simulink model "Energy_management_controller"  (R2014a)
settings: Solver=ode45  SolverMode=SingleTasking  StartTime=0.0  StopTime=10.0  RelTol=1e-3
libraries: fuzblock x1
(part 1 of 2)
settings Model: Creator=12730  LastModifiedBy=Administrator
settings OptimizationCC: BlockReduction=off  BooleanDataType=off  SimCompilerOptimization=off
settings DebuggingCC: SaveWithParameterizedLinksMsg=none  UnderspecifiedInitializationDetection=Classic  SignalResolutionControl=TryResolveAllWithWarning  SolverPrmCheckMsg=none  FrameProcessingCompatibilityMsg=error  StrictBusMsg=Warning
settings HardwareCC: TargetUnknown=on
settings RTWCC: RTWCompilerOptimization=off
settings ConfigComp: CovMetricSettings=dw  CovHtmlReporting=on  CovSaveCumulativeToWorkspaceVar=on  CovSaveSingleToWorkspaceVar=on  CovModelRefEnable=Off  CovExternalEMLEnable=off  CovSFcnEnable=off

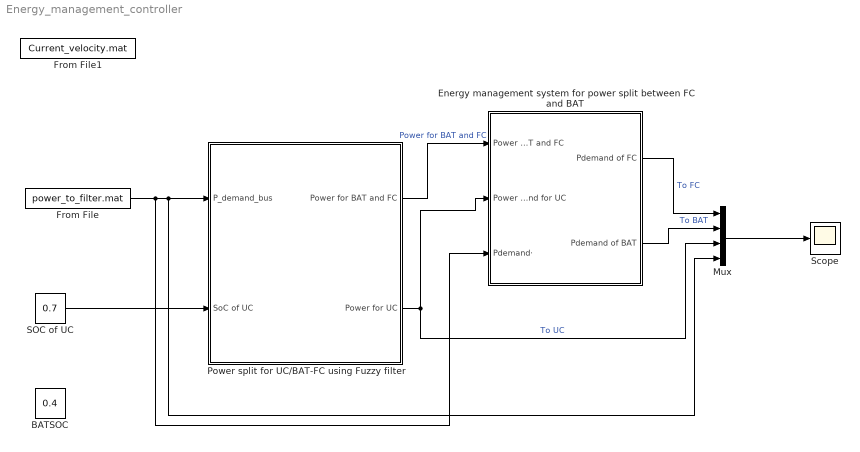
== system Energy_management_controller ==
  "BATSOC " : Constant  Value=0.4
  Energy management system for power split between FC and BAT : Subsystem
  From File : FromFile  FileName=power_to_filter.mat  SampleTime=0
  From File1 : FromFile  FileName=Current_velocity.mat  SampleTime=0
  Mux : Mux
  Power split for UC/BAT-FC using Fuzzy filter : Subsystem
  SOC of UC : Constant  Value=0.7
  Scope : Scope
  wires:
  From File/1 -> Power split for UC/BAT-FC using Fuzzy filter/1(P_demand_bus), Mux/4, Energy management system for power split between FC and BAT/3(Pdemand·)
  Power split for UC/BAT-FC using Fuzzy filter/1(Power for BAT and FC) -> Energy management system for power split between FC and BAT/1(Power demand for BAT and FC)  "Power for BAT and FC"
  Energy management system for power split between FC and BAT/2(Pdemand of BAT) -> Mux/2  "To BAT"
  Power split for UC/BAT-FC using Fuzzy filter/2(Power for UC) -> Energy management system for power split between FC and BAT/2(Power demand for UC), Mux/3  "To UC"
  SOC of UC/1 -> Power split for UC/BAT-FC using Fuzzy filter/2(SoC of UC)
  Mux/1 -> Scope/1
  Energy management system for power split between FC and BAT/1(Pdemand of FC) -> Mux/1  "To FC"

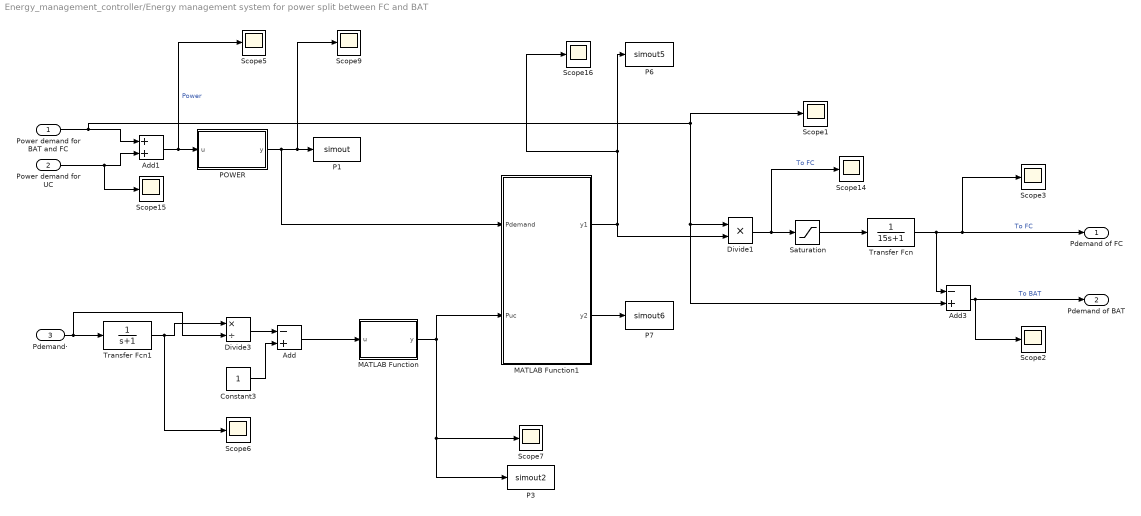
== system Energy_management_controller/Energy management system for power split between FC and BAT ==
  Power demand for BAT and FC : Inport
  Power demand for UC : Inport  Port=2
  Pdemand· : Inport  Port=3
  Add : Sum  Inputs=-+
  Add1 : Sum
  Add3 : Sum  Inputs=-+
  Constant3 : Constant
  Divide1 : Product  Inputs=**
  Divide3 : Product  Inputs=*/
  MATLAB Function : MATLAB Function  TreatAsAtomicUnit=on
  MATLAB Function1 : MATLAB Function  TreatAsAtomicUnit=on
  P1 : ToWorkspace  VariableName=simout  SaveFormat=Timeseries  SampleTime=-1
  P3 : ToWorkspace  VariableName=simout2  SaveFormat=Timeseries  SampleTime=-1
  P6 : ToWorkspace  VariableName=simout5  SaveFormat=Timeseries  SampleTime=-1
  P7 : ToWorkspace  VariableName=simout6  SaveFormat=Timeseries  SampleTime=-1
  POWER : MATLAB Function  TreatAsAtomicUnit=on
  Saturation : Saturate  UpperLimit=10000  LowerLimit=0.5
  Scope{1..3,5..7,9,14..16} (10 alike) : Scope
      Scope7 settings: SaveName=ScopeData3
  Transfer Fcn : TransferFcn  Denominator=[15 1]
  Transfer Fcn1 : TransferFcn  Denominator=[1 1]
  Pdemand of FC : Outport
  Pdemand of BAT : Outport  Port=2
  wires:
  Power demand for UC/1 -> Scope15/1, Add1/2
  Add1/1 -> POWER/1(u), Scope5/1  "Power"
  Add3/1 -> Scope2/1, Pdemand of BAT/1  "To BAT"
  Transfer Fcn/1 -> Add3/1, Pdemand of FC/1, Scope3/1  "To FC"
  Divide1/1 -> Scope14/1, Saturation/1  "To FC"
  Saturation/1 -> Transfer Fcn/1
  Pdemand·/1 -> Transfer Fcn1/1, Divide3/2
  Transfer Fcn1/1 -> Scope6/1, Divide3/1
  Divide3/1 -> Add/1
  Add/1 -> MATLAB Function/1(u)
  Constant3/1 -> Add/2
  MATLAB Function/1(y) -> P3/1, Scope7/1, MATLAB Function1/2(Puc)
  Power demand for BAT and FC/1 -> Add1/1, Add3/2, Divide1/1, Scope1/1
  MATLAB Function1/1(y1) -> Divide1/2, P6/1, Scope16/1
  MATLAB Function1/2(y2) -> P7/1
  POWER/1(y) -> MATLAB Function1/1(Pdemand), P1/1, Scope9/1

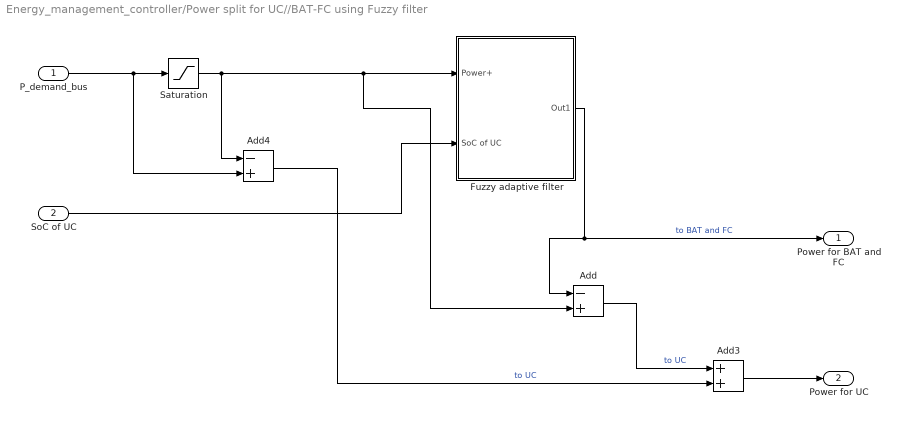
== system Energy_management_controller/Power split for UC//BAT-FC using Fuzzy filter ==
  P_demand_bus : Inport
  SoC of UC : Inport  Port=2
  Add : Sum  Inputs=-+
  Add3 : Sum
  Add4 : Sum  Inputs=-+
  Fuzzy adaptive filter : Subsystem
  Saturation : Saturate  UpperLimit=100000  LowerLimit=0
  Power for BAT and FC : Outport
  Power for UC : Outport  Port=2
  wires:
  SoC of UC/1 -> Fuzzy adaptive filter/2(SoC of UC)
  Fuzzy adaptive filter/1(Out1) -> Power for BAT and FC/1, Add/1  "to BAT and FC"
  P_demand_bus/1 -> Saturation/1, Add4/2
  Add/1 -> Add3/1  "to UC"
  Add4/1 -> Add3/2  "to UC"
  Add3/1 -> Power for UC/1
  Saturation/1 -> Add/2, Fuzzy adaptive filter/1(Power+), Add4/1

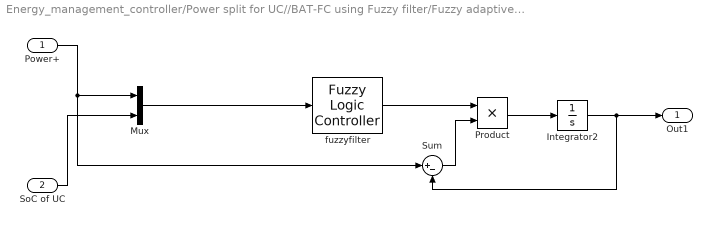
== system Energy_management_controller/Power split for UC//BAT-FC using Fuzzy filter/Fuzzy adaptive filter ==
  Power+ : Inport
  SoC of UC : Inport  Port=2
  Integrator2 : Integrator
  Mux : Mux  Inputs=2
  Product : Product
  Sum : Sum  Inputs=|+-
  fuzzyfilter : fuzblock/Fuzzy Logic  Controller  fis=['fuzzyfilter1']
  Out1 : Outport
  wires:
  Power+/1 -> Sum/1, Mux/1
  fuzzyfilter/1 -> Product/1
  Sum/1 -> Product/2
  Product/1 -> Integrator2/1
  Integrator2/1 -> Out1/1, Sum/2
  SoC of UC/1 -> Mux/2
  Mux/1 -> fuzzyfilter/1

== matlab function Energy_management_controller/Energy management system for power split between FC and BAT/MATLAB Function2 ==
  data: u input; y output
function y = fcn(u)
%#codegen

y = u;

== matlab function Energy_management_controller/Energy management system for power split between FC and BAT/POWER ==
  data: u input; y output
function y = fcn(u)
            n = floor(u);
            m = u - n;
            
     if m >= 0.25 &&m < 0.75
            m = 0.5;
            u = n + m;
        else if m < 0.25&& 0 <= m
            m = 0;
            u = n + m;
            else 
             m = 0;
             u = n + m + 1;
            end
      end
y = u;

== matlab function Energy_management_controller/Energy management system for power split between FC and BAT/MATLAB Function1 ==
  data: y1 output; Pdemand input; Puc input; y2 output
function [y1,y2] = fcn(Pdemand,Puc)

if Puc==0&&Pdemand>=0

    if Pdemand<=2.5
        P_FC = 0.1;
        P_BAT = 0.9;
        else if Pdemand>=3&&Pdemand<=9
            P_FC = 1;
            P_BAT = 0;
            else if Pdemand>=9.5&&Pdemand<=10
                P_FC = 0.95;
                P_BAT = 0.05;
                else if Pdemand>=10.5&&Pdemand<=12
                        P_FC = 0.65;
                        P_BAT = 0.35;
                    else if Pdemand>=12.5&&Pdemand<=14
                          P_FC = 0.6;
                        P_BAT = 0.4;
                        else if Pdemand>=14.5&&Pdemand<=15
                                  P_FC = 0.5;
                                P_BAT = 0.5;
                               else if Pdemand>=15.5&&Pdemand<=18.5
                                         P_FC = 0.4;
                                         P_BAT = 0.6;
%                                     else if Pdemand>=14.5&&Pdemand<=15
%                                           P_FC = 0.5;
%                                         P_BAT = 0.5;
%                                         else if Pdemand>=15&&Pdemand<=22.5
%                                                   P_FC = 0.5;
%                                                 P_BAT = 0.5;
                                            else 
                                                      P_FC = 0.35;
                                                    P_BAT = 0.65;
%                                          end
%                                         end
                                   end
                              end
                          end
                      end
                 end
            end
    end
else if Puc==0.2&&Pdemand>=0  
         
        if Pdemand>=0.5&&Pdemand<=4
                    P_FC = 0.2;
                    P_BAT = 0.8;
                else if Pdemand>=4.5&&Pdemand<=8.5
                            P_FC = 0.8;
                            P_BAT = 0.2;
                    else if Pdemand>=9&&Pdemand<=10
                                P_FC = 0.75;
                                P_BAT = 0.25;
                        else if Pdemand>=10.5&&Pdemand<=12
                                    P_FC = 0.5;
                                    P_BAT = 0.5;
                            else if Pdemand>=12.5&&Pdemand<=14
                                          P_FC = 0.55;
                                          P_BAT = 0.55;
                                else if Pdemand>=14.5&&Pdemand<=15
                                              P_FC = 0.45;
                                              P_BAT = 0.55;
                                       else if Pdemand>=15.5&&Pdemand<=18.5
                                                P_FC = 0.4;
                                                P_BAT = 0.6;
%                                             else if Pdemand>=12&&Pdemand<=14.5
%                                                       P_FC = 0.7;
%                                                       P_BAT = 0.3;
%                                                 else if Pdemand>=15&&Pdemand<=22.5
%                                                           P_FC = 0.5;
%                                                           P_BAT = 0.5;
                                                      else 
                                                              P_FC = 0.4;
                                                              P_BAT = 0.6;
%                                                     end
%                                                 end
                                           end
                                      end
                                  end
                              end
                         end
                    end
        end  
 else if Puc==0.4&&Pdemand>=0  
         
        if Pdemand>=0.5&&Pdemand<=5.5
                    P_FC = 0.1;
                    P_BAT = 0.9;
                else if Pdemand>=6&&Pdemand<=9
                            P_FC = 0.25;
                            P_BAT = 0.75;
                    else if Pdemand>=9.5&&Pdemand<=10.5
                                P_FC = 0.5;
                                P_BAT = 0.5;
                        else if Pdemand>=11&&Pdemand<=12
                                    P_FC = 0.3;
                                    P_BAT = 0.7;
                            else if Pdemand>=12.5&&Pdemand<=15
                                          P_FC = 0.45;
                                          P_BAT = 0.55;
                                else if Pdemand>=15.5&&Pdemand<=18.5
                                              P_FC = 0.4;
                                              P_BAT = 0.6;
%                                        else if Pdemand>=11&&Pdemand<=11.5
%                                                 P_FC = 0.8;
%                                                 P_BAT = 0.2;
%                                             else if Pdemand>=12&&Pdemand<=14.5
%                                                       P_FC = 0.7;
%                                                       P_BAT = 0.3;
%                                                 else if Pdemand>=15&&Pdemand<=22.5
%                                                           P_FC = 0.5;
%                                                           P_BAT = 0.5;
                                                      else 
                                                              P_FC = 0.35;
                                                              P_BAT = 0.65;
%                                                     end
%                                                 end
%                                            end
                                      end
                                  end
                              end
                         end
                    end
       end  
else if Puc==0.6&&Pdemand>=0  
         
        if Pdemand>=0.5&&Pdemand<=5.5
                    P_FC = 0.1;
                    P_BAT = 0.9;
                else if Pdemand>=6&&Pdemand<=9
                            P_FC = 0.25;
                            P_BAT = 0.75;
                    else if Pdemand>=9.5&&Pdemand<=10.5
                                P_FC = 0.35;
                                P_BAT = 0.65;
                        else if Pdemand>=11&&Pdemand<=12
                                    P_FC = 0.25;
                                    P_BAT = 0.75;
                            else if Pdemand>=12.5&&Pdemand<=18.5
                                          P_FC = 0.4;
                                          P_BAT = 0.6;
%                                 else if Pdemand>=15&&Pdemand<=22.5
%                                               P_FC = 0.5;
%                                               P_BAT = 0.5;
%                                        else if Pdemand>=11&&Pdemand<=11.5
%                                                 P_FC = 0.8;
%                                                 P_BAT = 0.2;
%                                             else if Pdemand>=12&&Pdemand<=14.5
%                                                       P_FC = 0.7;
%                                                       P_BAT = 0.3;
%                                                 else if Pdemand>=15&&Pdemand<=22.5
%                                                           P_FC = 0.5;
%                                                           P_BAT = 0.5;
                                                      else 
                                                              P_FC = 0.35;
                                                              P_BAT = 0.65;
%                                                     end
%                                                 end
%                                            end
%                                       end
                                  end
                              end
                         end
                    end
        end
 else if Puc==0.8&&Pdemand>=0  
         
        if Pdemand>=0.5&&Pdemand<=9.5
                    P_FC = 0.1;
                    P_BAT = 0.9;
                else if Pdemand>=10&&Pdemand<=10.5
                            P_FC = 0.05;
                            P_BAT = 0.95;
                    else if Pdemand>=11&&Pdemand<=12
                                P_FC = 0.2;
                                P_BAT = 0.8;
                        else if Pdemand>=12.5&&Pdemand<=13
                                    P_FC = 0.1;
                                    P_BAT = 0.9;
%                             else if Pdemand>=12&&Pdemand<=14.5
%                                           P_FC = 0.7;
%                                           P_BAT = 0.3;
%                                 else if Pdemand>=15&&Pdemand<=22.5
%                                               P_FC = 0.5;
%                                               P_BAT = 0.5;
%                                        else if Pdemand>=11&&Pdemand<=11.5
%                                                 P_FC = 0.8;
%                                                 P_BAT = 0.2;
%                                             else if Pdemand>=12&&Pdemand<=14.5
%                                                       P_FC = 0.7;
%                                                       P_BAT = 0.3;
%                                                 else if Pdemand>=15&&Pdemand<=22.5
%                                                           P_FC = 0.5;
%                                                           P_BAT = 0.5;
                                                      else 
                                                              P_FC = 0.2;
                                                              P_BAT = 0.8;
%                                                     end
%                                                 end
%                                            end
%                                       end
%                                   end
                              end
                         end
                    end
       end    
% else if BATsoc==0.4&&UCsoc==0.4&&Puc==0.25&&velocity>=0&&Pdemand>=0  
%          
%         if Pdemand>=0.5&&Pdemand<=4
%                     P_FC = 0.2;
%                     P_BAT = 0.8;
%                 else if Pdemand>=4.5&&Pdemand<=9
%                             P_FC = 1;
%                             P_BAT = 0;
%                     else if Pdemand>=9.5&&Pdemand<=10.5
%                                 P_FC = 0.9;
%                                 P_BAT = 0.1;
%                         else if Pdemand>=11&&Pdemand<=11.5
%                                     P_FC = 0.8;
%                                     P_BAT = 0.2;
%                             else if Pdemand>=12&&Pdemand<=14.5
%                                           P_FC = 0.7;
%                                           P_BAT = 0.3;
%                                 else if Pdemand>=15&&Pdemand<=22.5
%                                               P_FC = 0.5;
%                                               P_BAT = 0.5;
%                                        else if Pdemand>=11&&Pdemand<=11.5
%                                                 P_FC = 0.8;
%                                                 P_BAT = 0.2;
%                                             else if Pdemand>=12&&Pdemand<=14.5
%                                                       P_FC = 0.7;
%                                                       P_BAT = 0.3;
%                                                 else if Pdemand>=15&&Pdemand<=22.5
%                                                           P_FC = 0.5;
%                                                           P_BAT = 0.5;
%                                                       else 
%                                                               P_FC = 0.4;
%                                                               P_BAT = 0.6;
%                                                     end
%                                                 end
%                                            end
%                                       end
%                                   end
%                               end
%                          end
%                     end
%         end 
% else if BATsoc==0.4&&UCsoc==0.4&&Puc==0.3&&velocity>=0&&Pdemand>=0  
%          
%         if Pdemand>=0.5&&Pdemand<=4
%                     P_FC = 0.2;
%                     P_BAT = 0.8;
%                 else if Pdemand>=4.5&&Pdemand<=9
%                             P_FC = 1;
%                             P_BAT = 0;
%                     else if Pdemand>=9.5&&Pdemand<=10.5
%                                 P_FC = 0.9;
%                                 P_BAT = 0.1;
%                         else if Pdemand>=11&&Pdemand<=11.5
%                                     P_FC = 0.8;
%                                     P_BAT = 0.2;
%                             else if Pdemand>=12&&Pdemand<=14.5
%                                           P_FC = 0.7;
%                                           P_BAT = 0.3;
%                                 else if Pdemand>=15&&Pdemand<=22.5
%                                               P_FC = 0.5;
%                                               P_BAT = 0.5;
%                                        else if Pdemand>=11&&Pdemand<=11.5
%                                                 P_FC = 0.8;
%                                                 P_BAT = 0.2;
%                                             else if Pdemand>=12&&Pdemand<=14.5
%                                                       P_FC = 0.7;
%                                                       P_BAT = 0.3;
%                                                 else if Pdemand>=15&&Pdemand<=22.5
%                                                           P_FC = 0.5;
%                                                           P_BAT = 0.5;
%                                                       else 
%                                                               P_FC = 0.4;
%                                                               P_BAT = 0.6;
%                                                     end
%                                                 end
%                                            end
%                                       end
%                                   end
%                               end
%                          end
%                     end
%        end    
% else if BATsoc==0.4&&UCsoc==0.4&&Puc==0.35&&velocity>=0&&Pdemand>=0  
%          
%         if Pdemand>=0.5&&Pdemand<=4
%                     P_FC = 0.2;
%                     P_BAT = 0.8;
%                 else if Pdemand>=4.5&&Pdemand<=9
%                             P_FC = 1;
%                             P_BAT = 0;
%                     else if Pdemand>=9.5&&Pdemand<=10.5
%                                 P_FC = 0.9;
%                                 P_BAT = 0.1;
%                         else if Pdemand>=11&&Pdemand<=11.5
%                                     P_FC = 0.8;
%                                     P_BAT = 0.2;
%                             else if Pdemand>=12&&Pdemand<=14.5
%                                           P_FC = 0.7;
%                                           P_BAT = 0.3;
%                                 else if Pdemand>=15&&Pdemand<=22.5
%                                               P_FC = 0.5;
%                                               P_BAT = 0.5;
%                                        else if Pdemand>=11&&Pdemand<=11.5
%                                                 P_FC = 0.8;
%                                                 P_BAT = 0.2;
%                                             else if Pdemand>=12&&Pdemand<=14.5
%                                                       P_FC = 0.7;
%                                                       P_BAT = 0.3;
%                                                 else if Pdemand>=15&&Pdemand<=22.5
%                                                           P_FC = 0.5;
%                                                           P_BAT = 0.5;
%                                                       else 
%                                                               P_FC = 0.4;
%                                                               P_BAT = 0.6;
%                                                     end
%                                                 end
%                                            end
%                                       end
%                                   end
%                               end
%                          end
%                     end
%         end
%  else if BATsoc==0.4&&UCsoc==0.4&&Puc==0.4&&velocity>=0&&Pdemand>=0  
%          
%         if Pdemand>=0.5&&Pdemand<=4
%                     P_FC = 0.2;
%                     P_BAT = 0.8;
%                 else if Pdemand>=4.5&&Pdemand<=9
%                             P_FC = 1;
%                             P_BAT = 0;
%                     else if Pdemand>=9.5&&Pdemand<=10.5
%                                 P_FC = 0.9;
%                                 P_BAT = 0.1;
%                         else if Pdemand>=11&&Pdemand<=11.5
%                                     P_FC = 0.8;
%                                     P_BAT = 0.2;
%                             else if Pdemand>=12&&Pdemand<=14.5
%                                           P_FC = 0.7;
%                                           P_BAT = 0.3;
%                                 else if Pdemand>=15&&Pdemand<=22.5
%                                               P_FC = 0.5;
%                                               P_BAT = 0.5;
%                                        else if Pdemand>=11&&Pdemand<=11.5
%                                                 P_FC = 0.8;
%                                                 P_BAT = 0.2;
%                                             else if Pdemand>=12&&Pdemand<=14.5
%                                                       P_FC = 0.7;
%                                                       P_BAT = 0.3;
%                                                 else if Pdemand>=15&&Pdemand<=22.5
%                                                           P_FC = 0.5;
%                                                           P_BAT = 0.5;
%                                                       else 
%                                                               P_FC = 0.4;
%                                                               P_BAT = 0.6;
%                                                     end
%                                                 end
%                                            end
%                                       end
%                                   end
%                               end
%                          end
%                     end
%        end    
% else if BATsoc==0.4&&UCsoc==0.4&&Puc==0.45&&velocity>=0&&Pdemand>=0  
%          
%         if Pdemand>=0.5&&Pdemand<=4
%                     P_FC = 0.2;
%                     P_BAT = 0.8;
%                 else if Pdemand>=4.5&&Pdemand<=9
%                             P_FC = 1;
%                             P_BAT = 0;
%                     else if Pdemand>=9.5&&Pdemand<=10.5
%                                 P_FC = 0.9;
%                                 P_BAT = 0.1;
%                         else if Pdemand>=11&&Pdemand<=11.5
%                                     P_FC = 0.8;
%                                     P_BAT = 0.2;
%                             else if Pdemand>=12&&Pdemand<=14.5
%                                           P_FC = 0.7;
%                                           P_BAT = 0.3;
%                                 else if Pdemand>=15&&Pdemand<=22.5
%                                               P_FC = 0.5;
%                                               P_BAT = 0.5;
%                                        else if Pdemand>=11&&Pdemand<=11.5
%                                                 P_FC = 0.8;
%                                                 P_BAT = 0.2;
%                                             else if Pdemand>=12&&Pdemand<=14.5
%                                                       P_FC = 0.7;
%                                                       P_BAT = 0.3;
%                                                 else if Pdemand>=15&&Pdemand<=22.5
%                                                           P_FC = 0.5;
%                                                           P_BAT = 0.5;
%                                                       else 
%                                                               P_FC = 0.4;
%                                                               P_BAT = 0.6;
%                                                     end
%                                                 end
%                                            end
%                                       end
%                                   end
%                               end
%                          end
%                     end
%         end 
%  else if BATsoc==0.4&&UCsoc==0.4&&Puc==0.5&&velocity>=0&&Pdemand>=0  
%          
%         if Pdemand>=0.5&&Pdemand<=4
%                     P_FC = 0.2;
%                     P_BAT = 0.8;
%                 else if Pdemand>=4.5&&Pdemand<=9
%                             P_FC = 1;
%                             P_BAT = 0;
%                     else if Pdemand>=9.5&&Pdemand<=10.5
%                                 P_FC = 0.9;
%                                 P_BAT = 0.1;
%                         else if Pdemand>=11&&Pdemand<=11.5
%                                     P_FC = 0.8;
%                                     P_BAT = 0.2;
%                             else if Pdemand>=12&&Pdemand<=14.5
%                                           P_FC = 0.7;
%                                           P_BAT = 0.3;
%                                 else if Pdemand>=15&&Pdemand<=22.5
%                                               P_FC = 0.5;
%                                               P_BAT = 0.5;
%                                        else if Pdemand>=11&&Pdemand<=11.5
%                                                 P_FC = 0.8;
%                                                 P_BAT = 0.2;
%                                             else if Pdemand>=12&&Pdemand<=14.5
%                                                       P_FC = 0.7;
%                                                       P_BAT = 0.3;
%                                                 else if Pdemand>=15&&Pdemand<=22.5
%                                                           P_FC = 0.5;
%                                                           P_BAT = 0.5;
%                                                       else 
%                                                               P_FC = 0.4;
%                                                               P_BAT = 0.6;
%                                                     end
%                                                 end
%                                            end
%                                       end
%                                   end
%                               end
%                          end
%                     end
%        end    
% else if BATsoc==0.4&&UCsoc==0.4&&Puc==0.55&&velocity>=0&&Pdemand>=0  
%          
%         if Pdemand>=0.5&&Pdemand<=4
%                     P_FC = 0.2;
%                     P_BAT = 0.8;
%                 else if Pdemand>=4.5&&Pdemand<=9
%                             P_FC = 1;
%                             P_BAT = 0;
%                     else if Pdemand>=9.5&&Pdemand<=10.5
%                                 P_FC = 0.9;
%                                 P_BAT = 0.1;
%                         else if Pdemand>=11&&Pdemand<=11.5
%                                     P_FC = 0.8;
%                                     P_BAT = 0.2;
%                             else if Pdemand>=12&&Pdemand<=14.5
%                                           P_FC = 0.7;
%                                           P_BAT = 0.3;
%                                 else if Pdemand>=15&&Pdemand<=22.5
%                                               P_FC = 0.5;
%                                               P_BAT = 0.5;
%                                        else if Pdemand>=11&&Pdemand<=11.5
%                                                 P_FC = 0.8;
%                                                 P_BAT = 0.2;
%                                             else if Pdemand>=12&&Pdemand<=14.5
%                                                       P_FC = 0.7;
%                                                       P_BAT = 0.3;
%                                                 else if Pdemand>=15&&Pdemand<=22.5
%                                                           P_FC = 0.5;
%                                                           P_BAT = 0.5;
%                                                       else 
%                                                               P_FC = 0.4;
%                                                               P_BAT = 0.6;
%                                                     end
%                                                 end
%                                            end
%                                       end
%                                   end
%                               end
%                          end
%                     end
%         end
%  else if BATsoc==0.4&&UCsoc==0.4&&Puc==0.6&&velocity>=0&&Pdemand>=0  
%          
%         if Pdemand>=0.5&&Pdemand<=4
%                     P_FC = 0.2;
%                     P_BAT = 0.8;
%                 else if Pdemand>=4.5&&Pdemand<=9
%                             P_FC = 1;
%                             P_BAT = 0;
%                     else if Pdemand>=9.5&&Pdemand<=10.5
%                                 P_FC = 0.9;
%                                 P_BAT = 0.1;
%                         else if Pdemand>=11&&Pdemand<=11.5
%                                     P_FC = 0.8;
%                                     P_BAT = 0.2;
%                             else if Pdemand>=12&&Pdemand<=14.5
%                                           P_FC = 0.7;
%                                           P_BAT = 0.3;
%                                 else if Pdemand>=15&&Pdemand<=22.5
%                                               P_FC = 0.5;
%                                               P_BAT = 0.5;
%                                        else if Pdemand>=11&&Pdemand<=11.5
%                                                 P_FC = 0.8;
%                                                 P_BAT = 0.2;
%                                             else if Pdemand>=12&&Pdemand<=14.5
%                                                       P_FC = 0.7;
%                                                       P_BAT = 0.3;
%                                                 else if Pdemand>=15&&Pdemand<=22.5
%                                                           P_FC = 0.5;
%                                                           P_BAT = 0.5;
%                                                       else 
%                                                               P_FC = 0.4;
%                                                               P_BAT = 0.6;
%                                                     end
%                                                 end
%                                            end
%                                       end
%                                   end
%                               end
%                          end
%                     end
%        end    
% else if BATsoc==0.4&&UCsoc==0.4&&Puc==0.65&&velocity>=0&&Pdemand>=0  
%          
%         if Pdemand>=0.5&&Pdemand<=4
%                     P_FC = 0.2;
%                     P_BAT = 0.8;
%                 else if Pdemand>=4.5&&Pdemand<=9
%                             P_FC = 1;
%                             P_BAT = 0;
%                     else if Pdemand>=9.5&&Pdemand<=10.5
%                                 P_FC = 0.9;
%                                 P_BAT = 0.1;
%                         else if Pdemand>=11&&Pdemand<=11.5
%                                     P_FC = 0.8;
%                                     P_BAT = 0.2;
%                             else if Pdemand>=12&&Pdemand<=14.5
%                                           P_FC = 0.7;
%                                           P_BAT = 0.3;
%                                 else if Pdemand>=15&&Pdemand<=22.5
%                                               P_FC = 0.5;
%                                               P_BAT = 0.5;
%                                        else if Pdemand>=11&&Pdemand<=11.5
%                                                 P_FC = 0.8;
%                                                 P_BAT = 0.2;
%                                             else if Pdemand>=12&&Pdemand<=14.5
%                                                       P_FC = 0.7;
%                                                       P_BAT = 0.3;
%                                                 else if Pdemand>=15&&Pdemand<=22.5
%                                                           P_FC = 0.5;
%                                                           P_BAT = 0.5;
%                                                       else 
%                                                               P_FC = 0.4;
%                                                               P_BAT = 0.6;
%                                                     end
%                                                 end
%                                            end
%                                       end
%                                   end
%                               end
%                          end
%                     end
%         end 
% else if BATsoc==0.4&&UCsoc==0.4&&Puc==0.7&&velocity>=0&&Pdemand>=0  
%          
%         if Pdemand>=0.5&&Pdemand<=4
%                     P_FC = 0.2;
%                     P_BAT = 0.8;
%                 else if Pdemand>=4.5&&Pdemand<=9
%                             P_FC = 1;
%                             P_BAT = 0;
%                     else if Pdemand>=9.5&&Pdemand<=10.5
%                                 P_FC = 0.9;
%                                 P_BAT = 0.1;
%                         else if Pdemand>=11&&Pdemand<=11.5
%                                     P_FC = 0.8;
%                                     P_BAT = 0.2;
%                             else if Pdemand>=12&&Pdemand<=14.5
%                                           P_FC = 0.7;
%                                           P_BAT = 0.3;
%                                 else if Pdemand>=15&&Pdemand<=22.5
%                                               P_FC = 0.5;
%                                               P_BAT = 0.5;
%                                        else if Pdemand>=11&&Pdemand<=11.5
%                                                 P_FC = 0.8;
%                                                 P_BAT = 0.2;
%                                             else if Pdemand>=12&&Pdemand<=14.5
%                                                       P_FC = 0.7;
%                                                       P_BAT = 0.3;
%                                                 else if Pdemand>=15&&Pdemand<=22.5
%                                                           P_FC = 0.5;
%                                                           P_BAT = 0.5;
%                                                       else 
%                                                               P_FC = 0.4;
%                                                               P_BAT = 0.6;
%                                                     end
%                                                 end
%                                            end
%                                       end
%                                   end
%                               end
%                          end
%                     end
%        end    
% else if BATsoc==0.4&&UCsoc==0.4&&Puc==0.75&&velocity>=0&&Pdemand>=0  
%          
%         if Pdemand>=0.5&&Pdemand<=4
%                     P_FC = 0.2;
%                     P_BAT = 0.8;
%                 else if Pdemand>=4.5&&Pdemand<=9
%                             P_FC = 1;
%                             P_BAT = 0;
%                     else if Pdemand>=9.5&&Pdemand<=10.5
%                                 P_FC = 0.9;
%                                 P_BAT = 0.1;
%                         else if Pdemand>=11&&Pdemand<=11.5
%                                     P_FC = 0.8;
%                                     P_BAT = 0.2;
%                             else if Pdemand>=12&&Pdemand<=14.5
%                                           P_FC = 0.7;
%                                           P_BAT = 0.3;
%                                 else if Pdemand>=15&&Pdemand<=22.5
%                                               P_FC = 0.5;
%                                               P_BAT = 0.5;
%                                        else if Pdemand>=11&&Pdemand<=11.5
%                                                 P_FC = 0.8;
%                                                 P_BAT = 0.2;
%                                             else if Pdemand>=12&&Pdemand<=14.5
%                                                       P_FC = 0.7;
%                                                       P_BAT = 0.3;
%                                                 else if Pdemand>=15&&Pdemand<=22.5
%                                                           P_FC = 0.5;
%                                                           P_BAT = 0.5;
%                                                       else 
%                                                               P_FC = 0.4;
%                                                               P_BAT = 0.6;
%                                                     end
%                                                 end
%                                            end
%                                       end
%                                   end
%                               end
%                          end
%                     end
%         end
%  else if BATsoc==0.4&&UCsoc==0.4&&Puc==0.8&&velocity>=0&&Pdemand>=0  
%          
%         if Pdemand>=0.5&&Pdemand<=4
%                     P_FC = 0.2;
%                     P_BAT = 0.8;
%                 else if Pdemand>=4.5&&Pdemand<=9
%                             P_FC = 1;
%                             P_BAT = 0;
%                     else if Pdemand>=9.5&&Pdemand<=10.5
%                                 P_FC = 0.9;
%                                 P_BAT = 0.1;
%                         else if Pdemand>=11&&Pdemand<=11.5
%                                     P_FC = 0.8;
%                                     P_BAT = 0.2;
%                             else if Pdemand>=12&&Pdemand<=14.5
%                                           P_FC = 0.7;
%                                           P_BAT = 0.3;
%                                 else if Pdemand>=15&&Pdemand<=22.5
%                                               P_FC = 0.5;
%                                               P_BAT = 0.5;
%                                        else if Pdemand>=11&&Pdemand<=11.5
%                                                 P_FC = 0.8;
%                                                 P_BAT = 0.2;
%                                             else if Pdemand>=12&&Pdemand<=14.5
%                                                       P_FC = 0.7;
%                                                       P_BAT = 0.3;
%                                                 else if Pdemand>=15&&Pdemand<=22.5
%                                                           P_FC = 0.5;
%                                                           P_BAT = 0.5;
%                                                       else 
%                                                               P_FC = 0.4;
%                                                               P_BAT = 0.6;
%                                                     end
%                                                 end
%                                            end
%                                       end
%                                   end
%                               end
%                          end
%                     end
%        end    
% else if BATsoc==0.4&&UCsoc==0.4&&Puc==0.85&&velocity>=0&&Pdemand>=0  
%          
%         if Pdemand>=0.5&&Pdemand<=4
%                     P_FC = 0.2;
%                     P_BAT = 0.8;
%                 else if Pdemand>=4.5&&Pdemand<=9
%                             P_FC = 1;
%                             P_BAT = 0;
%                     else if Pdemand>=9.5&&Pdemand<=10.5
%                                 P_FC = 0.9;
%                                 P_BAT = 0.1;
%                         else if Pdemand>=11&&Pdemand<=11.5
%                                     P_FC = 0.8;
%                                     P_BAT = 0.2;
%                             else if Pdemand>=12&&Pdemand<=14.5
%                                           P_FC = 0.7;
%                                           P_BAT = 0.3;
%                                 else if Pdemand>=15&&Pdemand<=22.5
%                                               P_FC = 0.5;
%                                               P_BAT = 0.5;
%                                        else if Pdemand>=11&&Pdemand<=11.5
%                                                 P_FC = 0.8;
%                                                 P_BAT = 0.2;
%                                             else if Pdemand>=12&&Pdemand<=14.5
%                                                       P_FC = 0.7;
%                                                       P_BAT = 0.3;
%                                                 else if Pdemand>=15&&Pdemand<=22.5
%                                                           P_FC = 0.5;
%                                                           P_BAT = 0.5;
%                                                       else 
%                                                               P_FC = 0.4;
%                                                               P_BAT = 0.6;
%                                                     end
%                                                 end
%                                            end
%                                       end
%                                   end
%                               end
%                          end
%                     end
%         end
%   else if BATsoc==0.4&&UCsoc==0.4&&Puc==0.9&&velocity>=0&&Pdemand>=0  
%          
%         if Pdemand>=0.5&&Pdemand<=4
%                     P_FC = 0.2;
%                     P_BAT = 0.8;
%                 else if Pdemand>=4.5&&Pdemand<=9
%                             P_FC = 1;
%                             P_BAT = 0;
%                     else if Pdemand>=9.5&&Pdemand<=10.5
%                                 P_FC = 0.9;
%                                 P_BAT = 0.1;
%                         else if Pdemand>=11&&Pdemand<=11.5
%                                     P_FC = 0.8;
%                                     P_BAT = 0.2;
%                             else if Pdemand>=12&&Pdemand<=14.5
%                                           P_FC = 0.7;
%                                           P_BAT = 0.3;
%                                 else if Pdemand>=15&&Pdemand<=22.5
%                                               P_FC = 0.5;
%                                               P_BAT = 0.5;
%                                        else if Pdemand>=11&&Pdemand<=11.5
%                                                 P_FC = 0.8;
%                                                 P_BAT = 0.2;
%                                             else if Pdemand>=12&&Pdemand<=14.5
%                                                       P_FC = 0.7;
%                                                       P_BAT = 0.3;
%                                                 else if Pdemand>=15&&Pdemand<=22.5
%                                                           P_FC = 0.5;
%                                                           P_BAT = 0.5;
%                                                       else 
%                                                               P_FC = 0.4;
%                                                               P_BAT = 0.6;
%                                                     end
%                                                 end
%                                            end
%                                       end
%                                   end
%                               end
%                          end
%                     end
%        end    
% else if BATsoc==0.4&&UCsoc==0.4&&Puc==0.95&&velocity>=0&&Pdemand>=0  
%          
%         if Pdemand>=0.5&&Pdemand<=4
%                     P_FC = 0.2;
%                     P_BAT = 0.8;
%                 else if Pdemand>=4.5&&Pdemand<=9
%                             P_FC = 1;
%                             P_BAT = 0;
%                     else if Pdemand>=9.5&&Pdemand<=10.5
%                                 P_FC = 0.9;
%                                 P_BAT = 0.1;
%                         else if Pdemand>=11&&Pdemand<=11.5
%                                     P_FC = 0.8;
%                                     P_BAT = 0.2;
%                             else if Pdemand>=12&&Pdemand<=14.5
%                                           P_FC = 0.7;
%                                           P_BAT = 0.3;
%                                 else if Pdemand>=15&&Pdemand<=22.5
%                                               P_FC = 0.5;
%                                               P_BAT = 0.5;
%                                        else if Pdemand>=11&&Pdemand<=11.5
%                                                 P_FC = 0.8;
%                                                 P_BAT = 0.2;
%                                             else if Pdemand>=12&&Pdemand<=14.5
%                                                       P_FC = 0.7;
%                                                       P_BAT = 0.3;
%                                                 else if Pdemand>=15&&Pdemand<=22.5
%                                                           P_FC = 0.5;
%                                                           P_BAT = 0.5;
%                                                       else 
%                                                               P_FC = 0.4;
%                                                               P_BAT = 0.6;
%                                                     end
%                                                 end
%                                            end
%                                       end
%                                   end
%                               end
%                          end
%                     end
%         end      
 else
    P_FC = 0.4;
    P_BAT = 0.6;
%     end
%       end
%     end
%      end
%     end
%      end
%     end
%      end
%      end
%       end
%     end
%      end
%     end
%       end
%      end
     end 
    end
     end
    end
    
end   
  
y1 = P_FC;
y2 = P_BAT;
